simulink model "VAD_Top"  (R2016b)
settings: Solver=VariableStepAuto  StartTime=0.0  StopTime=100.0  RelTol=1e-3
undefined symbols (not defined in the file): get, magnitude
libraries: dspsnks4 x3, dspsigops x2, audiosources x1, dspstat3 x1, simulink x1, dspmathops x1, dspsrcs4 x1
settings Model: Creator=MizWong  LastModifiedBy=MizWong

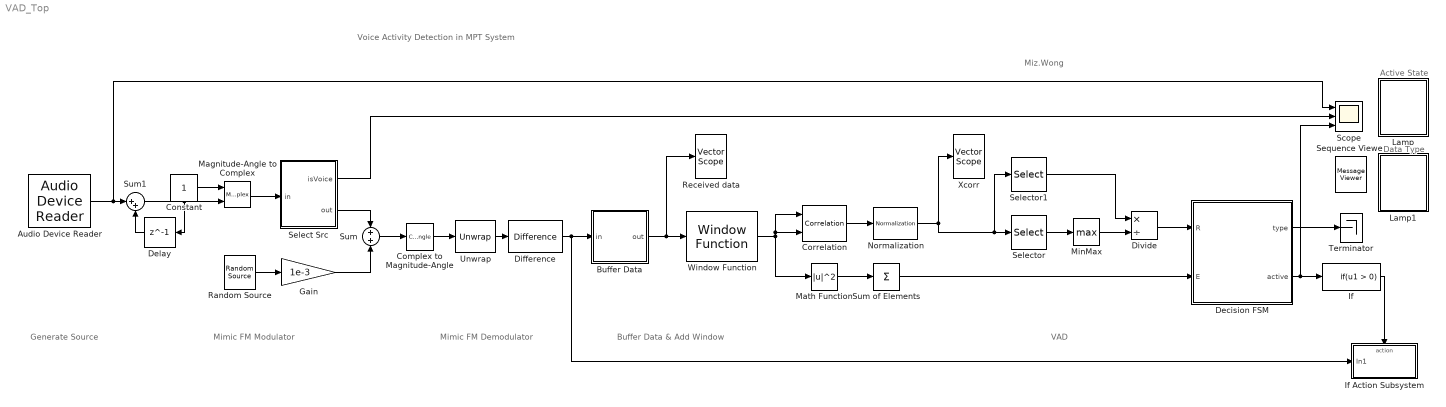
== system VAD_Top ==
  note: Data Type
  note: Active State
  note: Miz.Wong
  note: Voice Activity Detection in MPT System
  note: VAD
  note: Mimic FM Modulator
  note: Generate Source
  note: Mimic FM Demodulator
  note: Buffer Data & Add Window
  Audio Device Reader : audiosources/Audio Device Reader  Driver=DirectSound  Device=Default  SampleRate=8000  NumChannels=1  SamplesPerFrame=8000*0.03  BitDepth=16-bit integer  NumBuffers=10  DefaultInputChannelMapping=on  InputChannelMapping=1:2  OutputNumOverrunSamples=off  OutputDataType=double  DriverIdx=1  DeviceWarnFlag=''
  Buffer Data : Stateflow chart  TreatAsAtomicUnit=on
  Complex to Magnitude-Angle : ComplexToMagnitudeAngle  Output=Angle
  Constant : Constant
  Correlation : dspstat3/Correlation  domain=Time  roundingMode=Floor  overflowMode=off  outputDataTypeStr=Inherit: Same as accumulator  outputMin=[]  outputMax=[]  outputLastDataTypeStr=Inherit: Same as accumulator
  Decision FSM : Stateflow chart  TreatAsAtomicUnit=on
  Delay : Delay  DelayLength=1
  Difference : simulink/Discrete/Difference  ICPrevInput=0.0  OutMin=[]  OutMax=[]  OutDataType=fixdt(1, 16)  OutScaling=2^-10  DoSatur=off
  Divide : Product  Inputs=*/
  Gain : Gain  Gain=1e-3
  If : If  ShowElse=off
  If Action Subsystem : Subsystem  TreatAsAtomicUnit=on
  Lamp : Subsystem  DialogController=hmiCreateDDGDialog  IsWebBlock=on  mask(MWDashboardBlock){webBlockId=d8403fd5-788a-4616-9e22-623a4af549df, webBlockType=lamp, ShowInLibBrowser=on, ShowInitialText=on, HMISrcModelName=VAD_Top2}
      mask prompts: webBlockType "WebBlock Type"; HMISrcModelName "Source Model"
      mask help: SimulinkHMI:dialogs:LampDialogDesc
      mask Help: helpview([docroot '/mapfiles/simulink.map'], 'hmi_lamp')
      mask Display:
      | if strcmp(get_param(bdroot(gcb),'BlockDiagramType'), 'library')
      |     image([(matlabroot) '/toolbox/simulink/hmi/icons/Lamp.png']);
      | end
  Lamp1 : Subsystem  DialogController=hmiCreateDDGDialog  IsWebBlock=on  mask(MWDashboardBlock){webBlockId=551a018b-8965-429e-8f17-ffe41a7b2109, webBlockType=lamp, ShowInLibBrowser=on, ShowInitialText=on, HMISrcModelName=VAD_Top2}
      mask prompts: webBlockType "WebBlock Type"; HMISrcModelName "Source Model"
      mask help: SimulinkHMI:dialogs:LampDialogDesc
      mask Help: helpview([docroot '/mapfiles/simulink.map'], 'hmi_lamp')
      mask Display:
      | if strcmp(get_param(bdroot(gcb),'BlockDiagramType'), 'library')
      |     image([(matlabroot) '/toolbox/simulink/hmi/icons/Lamp.png']);
      | end
  Magnitude-Angle to Complex : MagnitudeAngleToComplex
  Math Function : Math  Operator=magnitude^2  SaturateOnIntegerOverflow=on
  MinMax : MinMax  Function=max
  Normalization : dspmathops/Normalization  NormType=2-norm  Bias=1e-10  NormOver=Each column  Dimension=1  outputDataTypeStr=Inherit: Same as product output  outputLastDataTypeStr=Inherit: Same as product output  outputMin=[]  outputMax=[]  accumDataTypeStr=Inherit: Same as product output  accumLastDataTypeStr=Inherit: Same as product output  roundingMode=Floor  overflowMode=off
  Random Source : dspsrcs4/Random Source  SrcType=Gaussian  NormMethod=Ziggurat  CltLength=12  MinVal=-1e-3  MaxVal=1e-3  MeanVal=0  VarVal=1  RepMode=Not repeatable  rawSeed=1  IsInherit=off  SampMode=Discrete  SampTime=1/8e3  SampFrame=8e3*0.03  DataType=Double  OutComplex=Complex  OutputFrames=off
  Received data : dspsnks4/Vector Scope  ScopeProperties=on  Domain=Time  HorizSpan=1  DisplayProperties=off  AxisGrid=on  Memory=off  FrameNumber=on  AxisLegend=off  AxisZoom=off  OpenScopeAtSimStart=on  OpenScopeImmediately=off  FigPos=get(0,'defaultfigureposition')-[300 0 0 0]  AxisProperties=off  XUnits=Hertz  XRange=[0...Fs/2]  InheritXIncr=on  XIncr=1  XLabel=Time  XLimit=Auto  XMin=0  XMax=1  XStart=0  YUnits=dB  YLabel=Amplitude  LineProperties=off  XAxisParamsVer=6.9
      settings: YMin=-10  YMax=10
  Scope : Scope  NumInputPorts=3
  Select Src : Stateflow chart  TreatAsAtomicUnit=on
  Selector : Selector  InputPortWidth=1439  IndexOptions=Index vector (dialog)  Indices=[721+10:1439]  OutputSizes=1
  Selector1 : Selector  InputPortWidth=1439  IndexOptions=Index vector (dialog)  Indices=720  OutputSizes=1
  Sequence Viewer : MessageViewer
  Sum : Sum  Inputs=+|+
  Sum of Elements : Sum  Inputs=+
  Sum1 : Sum  Inputs=|++
  Terminator : Terminator
  Unwrap : dspsigops/Unwrap  tol=pi  running=off
  Window Function : dspsigops/Window Function  winmode=Apply window to input  wintype=Hamming  sampmode=Discrete  samptime=1/8e3  N=720  Rs=50  beta=10  winsamp=Symmetric  UserWindow=hamming  OptParams=off  UserParams={'symmetric'}  dataType=double  isSigned=on  wordLen=16  udDataType=sfix(16)  fracBitsMode=Best precision  numFracBits=15  roundingMode=Floor  overflowMode=off  numSidelobes=4  sidelobeLevel=-30
  Xcorr : dspsnks4/Vector Scope  ScopeProperties=on  Domain=Time  HorizSpan=1  DisplayProperties=off  AxisGrid=on  Memory=off  FrameNumber=on  AxisLegend=off  AxisZoom=off  OpenScopeAtSimStart=on  OpenScopeImmediately=off  FigPos=get(0,'defaultfigureposition')+[300 0 0 0]  AxisProperties=off  XUnits=Hertz  XRange=[0...Fs/2]  InheritXIncr=on  XIncr=1  XLabel=Time  XLimit=Auto  XMin=0  XMax=1  XStart=0  YUnits=dB  YLabel=Amplitude  LineProperties=off  XAxisParamsVer=6.9
      settings: YMin=-0.2  YMax=0.7
  wires:
  Delay/1 -> Sum1/2
  Sum1/1 -> Magnitude-Angle to Complex/2, Delay/1
  Constant/1 -> Magnitude-Angle to Complex/1
  Sum/1 -> Complex to Magnitude-Angle/1
  Unwrap/1 -> Difference/1
  Magnitude-Angle to Complex/1 -> Select Src/1(in)
  Select Src/2(out) -> Sum/1
  Random Source/1 -> Gain/1
  Gain/1 -> Sum/2
  Complex to Magnitude-Angle/1 -> Unwrap/1
  Buffer Data/1(out) -> Window Function/1, Received data/1
  Window Function/1 -> Correlation/1, Correlation/2, Math Function/1
  Correlation/1 -> Normalization/1
  Normalization/1 -> Xcorr/1, Selector1/1, Selector/1
  Math Function/1 -> Sum of Elements/1
  Selector/1 -> MinMax/1
  MinMax/1 -> Divide/2
  Selector1/1 -> Divide/1
  Divide/1 -> Decision FSM/1(R)
  Sum of Elements/1 -> Decision FSM/2(E)
  Select Src/1(isVoice) -> Scope/2
  Decision FSM/2(active) -> If/1, Scope/3
  Decision FSM/1(type) -> Terminator/1
  If/1 -> If Action Subsystem/Action
  Audio Device Reader/1 -> Scope/1, Sum1/1
  Difference/1 -> Buffer Data/1(in), If Action Subsystem/1(In1)

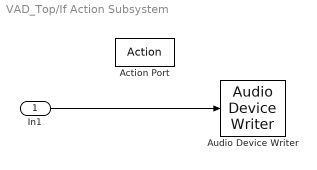
== system VAD_Top/If Action Subsystem ==
  In1 : Inport
  Action Port : ActionPort  ActionType=then
  Audio Device Writer : dspsnks4/Audio Device Writer  Driver=DirectSound  Device=Default  InheritSampleRate=off  SampleRate=8e3  BitDepth=16-bit integer  BufferSize=4096  NumBuffers=10  DefaultOutputChannelMapping=on  OutputChannelMapping=1:2  OutputNumUnderrunSamples=off  DriverIdx=1  DeviceWarnFlag=''
  wires:
  In1/1 -> Audio Device Writer/1

== system VAD_Top/Lamp ==

== system VAD_Top/Lamp1 ==

== stateflow chart VAD_Top/Buffer Data ==
  state data30ms
    entry:cnt=1;
    out = [zeros(8e3*0.03*2,1);in];
    buffer1=in;
  state data60ms
    entry:cnt=2;
    out = [zeros(8e3*0.03,1);buffer1;in];
    buffer2=[buffer1;in];
  state data90ms
    entry:out=[buffer2;in];
    buffer2=out(8e3*0.03+1:end);
    du:out=[buffer2;in];
    buffer2=out(8e3*0.03+1:end);
  (default) -> data30ms
  data30ms -> data60ms : [cnt==1]
  data60ms -> data90ms : [cnt==2]
  data: in input; out output size=720 [720..720]; buffer1 local; buffer2 local; cnt local =0

== stateflow chart VAD_Top/Decision FSM ==
  state Voice
    entry:type = 1;
    active = 1;
  state CH_Noise
    entry:type = 0;
    active = 0;
  state Soft_Noise
    entry: type = 2;
    active = 1;
  (junction 31) -> Voice [order 1] : [E>E_TH_L]
  Soft_Noise -> Voice [order 2] : [R<R_TH]
  Voice -> (junction 35) : [R>=R_TH]
  CH_Noise -> (junction 31) : [R<R_TH]
  (junction 31) -> CH_Noise [order 2] : [E<=E_TH_L]
  (default) -> CH_Noise
  (junction 35) -> CH_Noise [order 1] : [E>=E_TH_H]
  (junction 35) -> Soft_Noise [order 2] : [E<E_TH_H]
  Soft_Noise -> CH_Noise [order 1] : [E>=E_TH_H]
  data: R input; E input; type output =0; R_TH constant double =2.5; E_TH_L constant double =0.2; E_TH_H constant double =10; active output

== stateflow chart VAD_Top/Select Src ==
  state voice
    during: out = in;
    isVoice = 1;
  state noise
    during: out = zeros(8000*0.03,1);
    isVoice = 0;
  voice -> noise : [after(5,sec)]
  (default) -> voice
  noise -> voice : [after(1,sec)]
  data: isVoice output; in input; out output
